simulink model "EPT"  (R2019b)
settings: Solver=FixedStepDiscrete  StartTime=0.0  StopTime=5  FixedStep=0.005  RelTol=1e-3  EnableMultiTasking=on
PreLoadFcn:
  | try, model_open; catch, disp('Error occurred while executing model pre-load callback: model_open.m'); disp('Please assure that the MATLAB working directory is set to the model directory before opening.'); end
InitFcn:
  | try, model_open; catch, end
undefined symbols (not defined in the file or in its folder): Bridge, GCM, H, ln, raptor_get_param_eval, raptor_get_safe_string, raptor_xcp_function
libraries: Raptor_lib x2810, simulink x374, hdlsllib x19
(part 40 of 45)

== system EPT/Foreground_TimeBase_5ms/CAN/CAN3_exec/PWCU_GENERATOR/PWCU/PWCU3_Tx3/Convert_Data2Byte ==
  Data : Inport
  Factor : Inport  Port=2
  Offset : Inport  Port=3
  Add1 : Sum
  Bitwise Operator : simulink/Logic and Bit Operations/Bitwise Operator  logicop=AND  UseBitMask=on  BitMask=bin2dec('1111111100000000')  BitMaskRealWorld=Stored Integer
  Bitwise Operator1 : simulink/Logic and Bit Operations/Bitwise Operator  logicop=AND  UseBitMask=on  BitMask=bin2dec('0000000011111111')  BitMaskRealWorld=Stored Integer
  Constant : Constant
  Data Type Conversion1 : DataTypeConversion  OutDataTypeStr=uint16
  Divide1 : Product  Inputs=*/
  Divide2 : Product  Inputs=**
  Shift Arithmetic : ArithShift  BitShiftNumber=8  BitShiftDirection=Right
  HighByte : Outport  VectorParamsAs1DForOutWhenUnconnected=off
  LowByte : Outport  Port=2  VectorParamsAs1DForOutWhenUnconnected=off
  wires:
  Constant/1 -> Divide1/1
  Divide1/1 -> Divide2/2
  Factor/1 -> Divide1/2
  Bitwise Operator/1 -> Shift Arithmetic/1
  Offset/1 -> Add1/2
  Shift Arithmetic/1 -> HighByte/1
  Bitwise Operator1/1 -> LowByte/1
  Data Type Conversion1/1 -> Bitwise Operator/1, Bitwise Operator1/1
  Add1/1 -> Divide2/1
  Data/1 -> Add1/1
  Divide2/1 -> Data Type Conversion1/1

== system EPT/Foreground_TimeBase_5ms/CAN/CAN3_exec/PWCU_GENERATOR/PWCU/PWCU3_Tx3/Convert_Data2Byte1 ==
  Data : Inport
  Factor : Inport  Port=2
  Offset : Inport  Port=3
  Add1 : Sum
  Bitwise Operator : simulink/Logic and Bit Operations/Bitwise Operator  logicop=AND  UseBitMask=on  BitMask=bin2dec('1111111100000000')  BitMaskRealWorld=Stored Integer
  Bitwise Operator1 : simulink/Logic and Bit Operations/Bitwise Operator  logicop=AND  UseBitMask=on  BitMask=bin2dec('0000000011111111')  BitMaskRealWorld=Stored Integer
  Constant : Constant
  Data Type Conversion1 : DataTypeConversion  OutDataTypeStr=uint16
  Divide1 : Product  Inputs=*/
  Divide2 : Product  Inputs=**
  Shift Arithmetic : ArithShift  BitShiftNumber=8  BitShiftDirection=Right
  HighByte : Outport  VectorParamsAs1DForOutWhenUnconnected=off
  LowByte : Outport  Port=2  VectorParamsAs1DForOutWhenUnconnected=off
  wires:
  Constant/1 -> Divide1/1
  Divide1/1 -> Divide2/2
  Factor/1 -> Divide1/2
  Bitwise Operator/1 -> Shift Arithmetic/1
  Offset/1 -> Add1/2
  Shift Arithmetic/1 -> HighByte/1
  Bitwise Operator1/1 -> LowByte/1
  Data Type Conversion1/1 -> Bitwise Operator/1, Bitwise Operator1/1
  Add1/1 -> Divide2/1
  Data/1 -> Add1/1
  Divide2/1 -> Data Type Conversion1/1

== system EPT/Foreground_TimeBase_5ms/CAN/CAN3_exec/PWCU_GENERATOR/PWCU/Subsystem/Cmd_PWCU_Current_PI  ==
  PWCU1_Cout : Inport
  PWCU2_Cout : Inport  Port=2
  PWCU3_Cout : Inport  Port=3
  Ipwcu1_cc_exp : Inport  Port=4
  Ipwcu2_cc_exp : Inport  Port=5
  Ipwcu3_cc_exp : Inport  Port=6
  Enable : EnablePort
  Constant : Constant  Value=-inf
  Demux : Demux  Outputs=3
  Mux : Mux  Inputs=3
  Product : Product
  Product1 : Product
  Saturation Dynamic1 : simulink/Discontinuities/Saturation Dynamic  OutMin=[]  OutMax=[]  OutDataTypeStr=Inherit: Same as second input  OutDataType=fixdt(1, 16)  OutScaling=2^-10  DoSatur=off
  Saturation Dynamic2 : simulink/Discontinuities/Saturation Dynamic  OutMin=[]  OutMax=[]  OutDataTypeStr=Inherit: Same as second input  OutDataType=fixdt(1, 16)  OutScaling=2^-10  DoSatur=off
  Sum : Sum  Inputs=+-
  Sum1 : Sum  Inputs=+++
  Sum2 : Sum  Inputs=+-
  Sum3 : Sum  Inputs=+-
  raptor_adjustment2 : Raptor_lib/Data Storage/raptor_adjustment  paramName='Cal_PWCU_PID_KP'  nameSource=Parameter  initValue=0.5  dataType=double  storage=Calibration  calDispType=Number  calEnum={'False', 'True'}  calGain=1.0  calOffset=0.0  calMax=inf  calMin=-inf  calFormat='-1'  calUnit=''  calHelp=''  calAccess=1  calFunction=raptor_xcp_function(gcb)  calDispHeaders=off  calColHeaders={'Col1' 'Col2' 'Col3'}  calRowHeaders={'Row1' 'Row2' 'Row3'}
      settings: SourceProductName=Raptor
  raptor_adjustment4 : Raptor_lib/Data Storage/raptor_adjustment  paramName='Cal_PWCU_PID_KI'  nameSource=Parameter  initValue=0.2  dataType=double  storage=Calibration  calDispType=Number  calEnum={'False', 'True'}  calGain=1.0  calOffset=0.0  calMax=inf  calMin=-inf  calFormat='-1'  calUnit=''  calHelp=''  calAccess=1  calFunction=raptor_xcp_function(gcb)  calDispHeaders=off  calColHeaders={'Col1' 'Col2' 'Col3'}  calRowHeaders={'Row1' 'Row2' 'Row3'}
      settings: SourceProductName=Raptor
  PWCU1_Cout_Cmd : Outport  VectorParamsAs1DForOutWhenUnconnected=off
  PWCU2_Cout_Cmd : Outport  Port=2  VectorParamsAs1DForOutWhenUnconnected=off
  PWCU3_Cout_Cmd : Outport  Port=3  VectorParamsAs1DForOutWhenUnconnected=off
  wires:
  Constant/1 -> Saturation Dynamic2/3, Saturation Dynamic1/3
  raptor_adjustment4/1 -> Saturation Dynamic2/1, Product1/1
  Product/1 -> Saturation Dynamic1/2
  Saturation Dynamic1/1 -> Sum1/1
  Saturation Dynamic2/1 -> Sum1/2
  PWCU1_Cout/1 -> Sum/2
  Ipwcu1_cc_exp/1 -> Sum/1
  Product1/1 -> Saturation Dynamic2/2
  raptor_adjustment2/1 -> Saturation Dynamic1/1, Product/1
  Ipwcu2_cc_exp/1 -> Sum2/1
  PWCU2_Cout/1 -> Sum2/2
  Ipwcu3_cc_exp/1 -> Sum3/1
  PWCU3_Cout/1 -> Sum3/2
  Sum/1 -> Mux/1
  Sum2/1 -> Mux/2
  Sum3/1 -> Mux/3
  Mux/1 -> Sum1/3, Product1/2, Product/2
  Demux/2 -> PWCU2_Cout_Cmd/1
  Demux/1 -> PWCU1_Cout_Cmd/1
  Demux/3 -> PWCU3_Cout_Cmd/1
  Sum1/1 -> Demux/1

== system EPT/Foreground_TimeBase_5ms/CAN/CAN3_exec/PWCU_GENERATOR/PWCU/Subsystem/CountTrigger2 ==
  Counter : Inport
  Constant1 : Constant  Value=0
  Constant3 : Constant
  CycleTrigger : Subsystem
  Switch : Switch  Threshold=1
  Unit Delay : UnitDelay  SampleTime=-1  HasFrameUpgradeWarning=on
  Tirgger : Outport  VectorParamsAs1DForOutWhenUnconnected=off
  wires:
  Switch/1 -> CycleTrigger/1(In1)
  Constant3/1 -> Switch/3
  Constant1/1 -> Switch/1
  Counter/1 -> CycleTrigger/2(In2)
  CycleTrigger/1(Trigger) -> Tirgger/1, Unit Delay/1
  Unit Delay/1 -> Switch/2

== system EPT/Foreground_TimeBase_5ms/CAN/CAN3_exec/PWCU_GENERATOR/PWCU/Subsystem/Latch3 ==
  Latch : Inport
  Reset : Inport  Port=2
  Switch1 : Switch  Criteria=u2 > Threshold
  Switch3 : Switch  Criteria=u2 > Threshold
  Unit Delay1 : UnitDelay  SampleTime=-1  HasFrameUpgradeWarning=on
  Output : Outport  VectorParamsAs1DForOutWhenUnconnected=off
  wires:
  Unit Delay1/1 -> Switch1/3
  Switch3/1 -> Output/1, Unit Delay1/1
  Reset/1 -> Switch3/2
  Latch/1 -> Switch1/1, Switch1/2
  Switch1/1 -> Switch3/3

== system EPT/Foreground_TimeBase_5ms/CAN/CAN3_exec/PWCU_GENERATOR/PWCU/Subsystem/Latch4 ==
  Latch : Inport
  Reset : Inport  Port=2
  Switch1 : Switch  Criteria=u2 > Threshold
  Switch3 : Switch  Criteria=u2 > Threshold
  Unit Delay1 : UnitDelay  SampleTime=-1  HasFrameUpgradeWarning=on
  Output : Outport  VectorParamsAs1DForOutWhenUnconnected=off
  wires:
  Switch1/1 -> Switch3/3
  Latch/1 -> Switch1/2, Switch1/1
  Reset/1 -> Switch3/2
  Switch3/1 -> Unit Delay1/1, Output/1
  Unit Delay1/1 -> Switch1/3

== system EPT/Foreground_TimeBase_5ms/CAN/CAN3_exec/PWCU_GENERATOR/PWCU/Subsystem/Latch5 ==
  Latch : Inport
  Reset : Inport  Port=2
  Switch1 : Switch  Criteria=u2 > Threshold
  Switch3 : Switch  Criteria=u2 > Threshold
  Unit Delay1 : UnitDelay  SampleTime=-1  HasFrameUpgradeWarning=on
  Output : Outport  VectorParamsAs1DForOutWhenUnconnected=off
  wires:
  Switch1/1 -> Switch3/3
  Latch/1 -> Switch1/2, Switch1/1
  Reset/1 -> Switch3/2
  Switch3/1 -> Unit Delay1/1, Output/1
  Unit Delay1/1 -> Switch1/3

== system EPT/Foreground_TimeBase_5ms/CAN/CAN3_exec/SEVCON_MCU /SEVCON_TX_0X210_20ms /Delay/CycleTrigger ==
  In1 : Inport
  In2 : Inport  Port=2
  Add : Sum
  Add2 : Sum  Inputs=+-
  Constant2 : Constant  Value=0
  Constant3 : Constant
  Data Type Conversion1 : DataTypeConversion
  Data Type Conversion2 : DataTypeConversion
  Relational Operator1 : RelationalOperator  OutDataTypeStr=boolean  RndMeth=Simplest
  Saturation : Saturate  UpperLimit=inf  LowerLimit=2
  Switch : Switch  Threshold=1
  Unit Delay : UnitDelay  SampleTime=-1  HasFrameUpgradeWarning=on
  Trigger : Outport  VectorParamsAs1DForOutWhenUnconnected=off
  wires:
  Constant3/1 -> Add2/2
  In2/1 -> Saturation/1
  Add2/1 -> Data Type Conversion1/1
  Data Type Conversion2/1 -> Switch/2, Add/2
  Constant2/1 -> Switch/3
  Data Type Conversion1/1 -> Relational Operator1/2
  Relational Operator1/1 -> Trigger/1
  Switch/1 -> Unit Delay/1, Relational Operator1/1
  Unit Delay/1 -> Add/1
  In1/1 -> Data Type Conversion2/1
  Add/1 -> Switch/1
  Saturation/1 -> Add2/1

== system EPT/Foreground_TimeBase_5ms/CAN/CAN3_exec/SEVCON_MCU /SEVCON_TX_0X210_20ms /Delay1/CycleTrigger ==
  In1 : Inport
  In2 : Inport  Port=2
  Add : Sum
  Add2 : Sum  Inputs=+-
  Constant2 : Constant  Value=0
  Constant3 : Constant
  Data Type Conversion1 : DataTypeConversion
  Data Type Conversion2 : DataTypeConversion
  Relational Operator1 : RelationalOperator  OutDataTypeStr=boolean  RndMeth=Simplest
  Saturation : Saturate  UpperLimit=inf  LowerLimit=2
  Switch : Switch  Threshold=1
  Unit Delay : UnitDelay  SampleTime=-1  HasFrameUpgradeWarning=on
  Trigger : Outport  VectorParamsAs1DForOutWhenUnconnected=off
  wires:
  Constant3/1 -> Add2/2
  In2/1 -> Saturation/1
  Add2/1 -> Data Type Conversion1/1
  Data Type Conversion2/1 -> Switch/2, Add/2
  Constant2/1 -> Switch/3
  Data Type Conversion1/1 -> Relational Operator1/2
  Relational Operator1/1 -> Trigger/1
  Switch/1 -> Unit Delay/1, Relational Operator1/1
  Unit Delay/1 -> Add/1
  In1/1 -> Data Type Conversion2/1
  Add/1 -> Switch/1
  Saturation/1 -> Add2/1

== system EPT/Foreground_TimeBase_5ms/CAN/CAN3_exec/SEVCON_MCU /SEVCON_TX_0X210_20ms /Delay3/CycleTrigger ==
  In1 : Inport
  In2 : Inport  Port=2
  Add : Sum
  Add2 : Sum  Inputs=+-
  Constant2 : Constant  Value=0
  Constant3 : Constant
  Data Type Conversion1 : DataTypeConversion
  Data Type Conversion2 : DataTypeConversion
  Relational Operator1 : RelationalOperator  OutDataTypeStr=boolean  RndMeth=Simplest
  Saturation : Saturate  UpperLimit=inf  LowerLimit=2
  Switch : Switch  Threshold=1
  Unit Delay : UnitDelay  SampleTime=-1  HasFrameUpgradeWarning=on
  Trigger : Outport  VectorParamsAs1DForOutWhenUnconnected=off
  wires:
  Saturation/1 -> Add2/1
  Add/1 -> Switch/1
  In1/1 -> Data Type Conversion2/1
  Unit Delay/1 -> Add/1
  Switch/1 -> Relational Operator1/1, Unit Delay/1
  Relational Operator1/1 -> Trigger/1
  Data Type Conversion1/1 -> Relational Operator1/2
  Constant2/1 -> Switch/3
  Data Type Conversion2/1 -> Add/2, Switch/2
  Add2/1 -> Data Type Conversion1/1
  In2/1 -> Saturation/1
  Constant3/1 -> Add2/2

== system EPT/Foreground_TimeBase_5ms/CAN/CAN3_exec/SWCU/EPT to SWCU Enable Control/Delay/CycleTrigger ==
  In1 : Inport
  In2 : Inport  Port=2
  Add : Sum
  Add1 : Sum
  Add2 : Sum  Inputs=+-
  Constant1 : Constant
  Constant2 : Constant  Value=0
  Constant3 : Constant
  Data Type Conversion1 : DataTypeConversion
  Data Type Conversion2 : DataTypeConversion
  Display : Display
  Relational Operator1 : RelationalOperator  OutDataTypeStr=boolean  RndMeth=Simplest
  Saturation : Saturate  UpperLimit=inf  LowerLimit=2
  Scope : Scope
  Scope1 : Scope
  Scope2 : Scope
  Switch : Switch  Threshold=1
  Unit Delay : UnitDelay  SampleTime=-1  HasFrameUpgradeWarning=on
  Unit Delay1 : UnitDelay  SampleTime=-1  HasFrameUpgradeWarning=on
  Trigger : Outport  VectorParamsAs1DForOutWhenUnconnected=off
  wires:
  Saturation/1 -> Add2/1
  Add/1 -> Switch/1
  In1/1 -> Data Type Conversion2/1
  Unit Delay/1 -> Add/1
  Switch/1 -> Relational Operator1/1, Scope1/1, Unit Delay/1
  Add1/1 -> Scope/1, Unit Delay1/1, Display/1
  Unit Delay1/1 -> Add1/1
  Constant1/1 -> Add1/2
  Relational Operator1/1 -> Scope2/1, Trigger/1
  Data Type Conversion1/1 -> Relational Operator1/2
  Constant2/1 -> Switch/3
  Data Type Conversion2/1 -> Add/2, Switch/2
  Add2/1 -> Data Type Conversion1/1
  In2/1 -> Saturation/1
  Constant3/1 -> Add2/2

== system EPT/Foreground_TimeBase_5ms/CHG//DCHG_PW_Control/Coulomb Counting Algorithm/Coulomb Counting Algorithm/20ms/CountTrigger3/CycleTrigger ==
  In1 : Inport
  In2 : Inport  Port=2
  Add : Sum
  Add2 : Sum  Inputs=+-
  Constant2 : Constant  Value=0
  Constant3 : Constant
  Data Type Conversion1 : DataTypeConversion
  Data Type Conversion2 : DataTypeConversion
  Relational Operator1 : RelationalOperator  OutDataTypeStr=boolean  RndMeth=Simplest
  Scope1 : Scope
  Scope2 : Scope
  Switch : Switch  Threshold=1
  Unit Delay : UnitDelay  SampleTime=-1  HasFrameUpgradeWarning=on
  Trigger : Outport  VectorParamsAs1DForOutWhenUnconnected=off
  wires:
  Constant3/1 -> Add2/2
  In2/1 -> Add2/1
  Add2/1 -> Data Type Conversion1/1
  Data Type Conversion2/1 -> Switch/2, Add/2
  Constant2/1 -> Switch/3
  Data Type Conversion1/1 -> Relational Operator1/2
  Relational Operator1/1 -> Trigger/1, Scope2/1
  Switch/1 -> Unit Delay/1, Scope1/1, Relational Operator1/1
  Unit Delay/1 -> Add/1
  In1/1 -> Data Type Conversion2/1
  Add/1 -> Switch/1

== system EPT/Foreground_TimeBase_5ms/CHG//DCHG_PW_Control/Coulomb Counting Algorithm/WH /20ms/CountTrigger3/CycleTrigger ==
  In1 : Inport
  In2 : Inport  Port=2
  Add : Sum
  Add2 : Sum  Inputs=+-
  Constant2 : Constant  Value=0
  Constant3 : Constant
  Data Type Conversion1 : DataTypeConversion
  Data Type Conversion2 : DataTypeConversion
  Relational Operator1 : RelationalOperator  OutDataTypeStr=boolean  RndMeth=Simplest
  Scope1 : Scope
  Scope2 : Scope
  Switch : Switch  Threshold=1
  Unit Delay : UnitDelay  SampleTime=-1  HasFrameUpgradeWarning=on
  Trigger : Outport  VectorParamsAs1DForOutWhenUnconnected=off
  wires:
  Add/1 -> Switch/1
  In1/1 -> Data Type Conversion2/1
  Unit Delay/1 -> Add/1
  Switch/1 -> Relational Operator1/1, Scope1/1, Unit Delay/1
  Relational Operator1/1 -> Scope2/1, Trigger/1
  Data Type Conversion1/1 -> Relational Operator1/2
  Constant2/1 -> Switch/3
  Data Type Conversion2/1 -> Add/2, Switch/2
  Add2/1 -> Data Type Conversion1/1
  In2/1 -> Add2/1
  Constant3/1 -> Add2/2

== system EPT/Foreground_TimeBase_5ms/CHG//DCHG_PW_Control/Enhanced Coulomb Counting Algorithm/Coulomb Counting/20ms/CountTrigger3/CycleTrigger ==
  In1 : Inport
  In2 : Inport  Port=2
  Add : Sum
  Add2 : Sum  Inputs=+-
  Constant2 : Constant  Value=0
  Constant3 : Constant
  Data Type Conversion1 : DataTypeConversion
  Data Type Conversion2 : DataTypeConversion
  Relational Operator1 : RelationalOperator  OutDataTypeStr=boolean  RndMeth=Simplest
  Scope1 : Scope
  Scope2 : Scope
  Switch : Switch  Threshold=1
  Unit Delay : UnitDelay  SampleTime=-1  HasFrameUpgradeWarning=on
  Trigger : Outport  VectorParamsAs1DForOutWhenUnconnected=off
  wires:
  Add/1 -> Switch/1
  In1/1 -> Data Type Conversion2/1
  Unit Delay/1 -> Add/1
  Switch/1 -> Relational Operator1/1, Scope1/1, Unit Delay/1
  Relational Operator1/1 -> Scope2/1, Trigger/1
  Data Type Conversion1/1 -> Relational Operator1/2
  Constant2/1 -> Switch/3
  Data Type Conversion2/1 -> Add/2, Switch/2
  Add2/1 -> Data Type Conversion1/1
  In2/1 -> Add2/1
  Constant3/1 -> Add2/2

== system EPT/Foreground_TimeBase_5ms/CHG//DCHG_PW_Control/Enhanced Coulomb Counting Algorithm Backup/Coulomb Counting1/20ms/CountTrigger3/CycleTrigger ==
  In1 : Inport
  In2 : Inport  Port=2
  Add : Sum
  Add2 : Sum  Inputs=+-
  Constant2 : Constant  Value=0
  Constant3 : Constant
  Data Type Conversion1 : DataTypeConversion
  Data Type Conversion2 : DataTypeConversion
  Relational Operator1 : RelationalOperator  OutDataTypeStr=boolean  RndMeth=Simplest
  Scope1 : Scope
  Scope2 : Scope
  Switch : Switch  Threshold=1
  Unit Delay : UnitDelay  SampleTime=-1  HasFrameUpgradeWarning=on
  Trigger : Outport  VectorParamsAs1DForOutWhenUnconnected=off
  wires:
  Constant3/1 -> Add2/2
  In2/1 -> Add2/1
  Add2/1 -> Data Type Conversion1/1
  Data Type Conversion2/1 -> Switch/2, Add/2
  Constant2/1 -> Switch/3
  Data Type Conversion1/1 -> Relational Operator1/2
  Relational Operator1/1 -> Trigger/1, Scope2/1
  Switch/1 -> Unit Delay/1, Scope1/1, Relational Operator1/1
  Unit Delay/1 -> Add/1
  In1/1 -> Data Type Conversion2/1
  Add/1 -> Switch/1

== system EPT/Foreground_TimeBase_5ms/E//W /BP-OBU_E//W/BP-OBU_E//W/BP-OBU_Fault_G4/Fault CMU CAN ID/Delay34 ==
  Condition : Inport
  TimeCount : Inport  Port=2
  Constant10 : Constant
  Constant11 : Constant  Value=0
  Constant8 : Constant  Value=0
  CycleTrigger : Subsystem
  Switch2 : Switch  Threshold=1
  Switch3 : Switch  Threshold=1
  Unit Delay1 : UnitDelay  SampleTime=-1  HasFrameUpgradeWarning=on
  Unit Delay2 : UnitDelay  SampleTime=-1  HasFrameUpgradeWarning=on
  Output : Outport  VectorParamsAs1DForOutWhenUnconnected=off
  wires:
  TimeCount/1 -> CycleTrigger/2(In2)
  Condition/1 -> Switch3/2
  CycleTrigger/1(Trigger) -> Switch2/2, Unit Delay1/1
  Constant8/1 -> Switch2/1
  Constant10/1 -> Switch2/3
  Switch3/1 -> CycleTrigger/1(In1)
  Constant11/1 -> Switch3/3
  Unit Delay2/1 -> Switch3/1
  Switch2/1 -> Unit Delay2/1
  Unit Delay1/1 -> Output/1

== system EPT/Foreground_TimeBase_5ms/E//W /BP-OBU_E//W/BP-OBU_E//W/BP-OBU_Fault_G4/Fault CMU CAN ID/Delay35 ==
  Condition : Inport
  TimeCount : Inport  Port=2
  Constant10 : Constant
  Constant11 : Constant  Value=0
  Constant8 : Constant  Value=0
  CycleTrigger : Subsystem
  Switch2 : Switch  Threshold=1
  Switch3 : Switch  Threshold=1
  Unit Delay1 : UnitDelay  SampleTime=-1  HasFrameUpgradeWarning=on
  Unit Delay2 : UnitDelay  SampleTime=-1  HasFrameUpgradeWarning=on
  Output : Outport  VectorParamsAs1DForOutWhenUnconnected=off
  wires:
  Unit Delay1/1 -> Output/1
  Switch2/1 -> Unit Delay2/1
  Unit Delay2/1 -> Switch3/1
  Constant11/1 -> Switch3/3
  Switch3/1 -> CycleTrigger/1(In1)
  Constant10/1 -> Switch2/3
  Constant8/1 -> Switch2/1
  CycleTrigger/1(Trigger) -> Unit Delay1/1, Switch2/2
  Condition/1 -> Switch3/2
  TimeCount/1 -> CycleTrigger/2(In2)

== system EPT/Foreground_TimeBase_5ms/E//W /BP-OBU_E//W/BP-OBU_E//W/BP-OBU_Fault_G4/Fault CMU CAN ID/Latch39 ==
  Latch : Inport
  Reset : Inport  Port=2
  Switch1 : Switch  Criteria=u2 > Threshold
  Switch3 : Switch  Criteria=u2 > Threshold
  Unit Delay1 : UnitDelay  SampleTime=-1  HasFrameUpgradeWarning=on
  Output : Outport  VectorParamsAs1DForOutWhenUnconnected=off
  wires:
  Unit Delay1/1 -> Switch1/3
  Switch3/1 -> Output/1, Unit Delay1/1
  Reset/1 -> Switch3/2
  Latch/1 -> Switch1/1, Switch1/2
  Switch1/1 -> Switch3/3

== system EPT/Foreground_TimeBase_5ms/E//W /BP-OBU_E//W/BP-OBU_E//W/BP-OBU_Fault_G4/Fault CMU CAN ID/Latch40 ==
  Latch : Inport
  Reset : Inport  Port=2
  Switch1 : Switch  Criteria=u2 > Threshold
  Switch3 : Switch  Criteria=u2 > Threshold
  Unit Delay1 : UnitDelay  SampleTime=-1  HasFrameUpgradeWarning=on
  Output : Outport  VectorParamsAs1DForOutWhenUnconnected=off
  wires:
  Switch1/1 -> Switch3/3
  Latch/1 -> Switch1/2, Switch1/1
  Reset/1 -> Switch3/2
  Switch3/1 -> Unit Delay1/1, Output/1
  Unit Delay1/1 -> Switch1/3

== system EPT/Foreground_TimeBase_5ms/E//W /BP-OBU_E//W/BP-OBU_E//W/BP-OBU_Warning//Fault_G1/Internal Res E//W/Delay4 ==
  Condition : Inport
  TimeCount : Inport  Port=2
  Constant10 : Constant
  Constant11 : Constant  Value=0
  Constant8 : Constant  Value=0
  CycleTrigger : Subsystem
  Switch2 : Switch  Threshold=1
  Switch3 : Switch  Threshold=1
  Unit Delay1 : UnitDelay  SampleTime=-1  HasFrameUpgradeWarning=on
  Unit Delay2 : UnitDelay  SampleTime=-1  HasFrameUpgradeWarning=on
  Output : Outport  VectorParamsAs1DForOutWhenUnconnected=off
  wires:
  TimeCount/1 -> CycleTrigger/2(In2)
  Condition/1 -> Switch3/2
  CycleTrigger/1(Trigger) -> Switch2/2, Unit Delay1/1
  Constant8/1 -> Switch2/1
  Constant10/1 -> Switch2/3
  Switch3/1 -> CycleTrigger/1(In1)
  Constant11/1 -> Switch3/3
  Unit Delay2/1 -> Switch3/1
  Switch2/1 -> Unit Delay2/1
  Unit Delay1/1 -> Output/1

== system EPT/Foreground_TimeBase_5ms/E//W /BP-OBU_E//W/BP-OBU_E//W/BP-OBU_Warning//Fault_G1/Internal Res E//W/Delay5 ==
  Condition : Inport
  TimeCount : Inport  Port=2
  Constant10 : Constant
  Constant11 : Constant  Value=0
  Constant8 : Constant  Value=0
  CycleTrigger : Subsystem
  Switch2 : Switch  Threshold=1
  Switch3 : Switch  Threshold=1
  Unit Delay1 : UnitDelay  SampleTime=-1  HasFrameUpgradeWarning=on
  Unit Delay2 : UnitDelay  SampleTime=-1  HasFrameUpgradeWarning=on
  Output : Outport  VectorParamsAs1DForOutWhenUnconnected=off
  wires:
  Unit Delay1/1 -> Output/1
  Switch2/1 -> Unit Delay2/1
  Unit Delay2/1 -> Switch3/1
  Constant11/1 -> Switch3/3
  Switch3/1 -> CycleTrigger/1(In1)
  Constant10/1 -> Switch2/3
  Constant8/1 -> Switch2/1
  CycleTrigger/1(Trigger) -> Unit Delay1/1, Switch2/2
  Condition/1 -> Switch3/2
  TimeCount/1 -> CycleTrigger/2(In2)

== system EPT/Foreground_TimeBase_5ms/E//W /BP-OBU_E//W/BP-OBU_E//W/BP-OBU_Warning//Fault_G1/Internal Res E//W/Delay6 ==
  Condition : Inport
  TimeCount : Inport  Port=2
  Constant10 : Constant
  Constant11 : Constant  Value=0
  Constant8 : Constant  Value=0
  CycleTrigger : Subsystem
  Switch2 : Switch  Threshold=1
  Switch3 : Switch  Threshold=1
  Unit Delay1 : UnitDelay  SampleTime=-1  HasFrameUpgradeWarning=on
  Unit Delay2 : UnitDelay  SampleTime=-1  HasFrameUpgradeWarning=on
  Output : Outport  VectorParamsAs1DForOutWhenUnconnected=off
  wires:
  TimeCount/1 -> CycleTrigger/2(In2)
  Condition/1 -> Switch3/2
  CycleTrigger/1(Trigger) -> Switch2/2, Unit Delay1/1
  Constant8/1 -> Switch2/1
  Constant10/1 -> Switch2/3
  Switch3/1 -> CycleTrigger/1(In1)
  Constant11/1 -> Switch3/3
  Unit Delay2/1 -> Switch3/1
  Switch2/1 -> Unit Delay2/1
  Unit Delay1/1 -> Output/1

== system EPT/Foreground_TimeBase_5ms/E//W /BP-OBU_E//W/BP-OBU_E//W/BP-OBU_Warning//Fault_G1/Internal Res E//W/Delay7 ==
  Condition : Inport
  TimeCount : Inport  Port=2
  Constant10 : Constant
  Constant11 : Constant  Value=0
  Constant8 : Constant  Value=0
  CycleTrigger : Subsystem
  Switch2 : Switch  Threshold=1
  Switch3 : Switch  Threshold=1
  Unit Delay1 : UnitDelay  SampleTime=-1  HasFrameUpgradeWarning=on
  Unit Delay2 : UnitDelay  SampleTime=-1  HasFrameUpgradeWarning=on
  Output : Outport  VectorParamsAs1DForOutWhenUnconnected=off
  wires:
  Unit Delay1/1 -> Output/1
  Switch2/1 -> Unit Delay2/1
  Unit Delay2/1 -> Switch3/1
  Constant11/1 -> Switch3/3
  Switch3/1 -> CycleTrigger/1(In1)
  Constant10/1 -> Switch2/3
  Constant8/1 -> Switch2/1
  CycleTrigger/1(Trigger) -> Unit Delay1/1, Switch2/2
  Condition/1 -> Switch3/2
  TimeCount/1 -> CycleTrigger/2(In2)

== system EPT/Foreground_TimeBase_5ms/E//W /BP-OBU_E//W/BP-OBU_E//W/BP-OBU_Warning//Fault_G1/Internal Res E//W/Delay8 ==
  Condition : Inport
  TimeCount : Inport  Port=2
  Constant10 : Constant
  Constant11 : Constant  Value=0
  Constant8 : Constant  Value=0
  CycleTrigger : Subsystem
  Switch2 : Switch  Threshold=1
  Switch3 : Switch  Threshold=1
  Unit Delay1 : UnitDelay  SampleTime=-1  HasFrameUpgradeWarning=on
  Unit Delay2 : UnitDelay  SampleTime=-1  HasFrameUpgradeWarning=on
  Output : Outport  VectorParamsAs1DForOutWhenUnconnected=off
  wires:
  TimeCount/1 -> CycleTrigger/2(In2)
  Condition/1 -> Switch3/2
  CycleTrigger/1(Trigger) -> Switch2/2, Unit Delay1/1
  Constant8/1 -> Switch2/1
  Constant10/1 -> Switch2/3
  Switch3/1 -> CycleTrigger/1(In1)
  Constant11/1 -> Switch3/3
  Unit Delay2/1 -> Switch3/1
  Switch2/1 -> Unit Delay2/1
  Unit Delay1/1 -> Output/1

== system EPT/Foreground_TimeBase_5ms/E//W /BP-OBU_E//W/BP-OBU_E//W/BP-OBU_Warning//Fault_G1/Internal Res E//W/Delay9 ==
  Condition : Inport
  TimeCount : Inport  Port=2
  Constant10 : Constant
  Constant11 : Constant  Value=0
  Constant8 : Constant  Value=0
  CycleTrigger : Subsystem
  Switch2 : Switch  Threshold=1
  Switch3 : Switch  Threshold=1
  Unit Delay1 : UnitDelay  SampleTime=-1  HasFrameUpgradeWarning=on
  Unit Delay2 : UnitDelay  SampleTime=-1  HasFrameUpgradeWarning=on
  Output : Outport  VectorParamsAs1DForOutWhenUnconnected=off
  wires:
  Unit Delay1/1 -> Output/1
  Switch2/1 -> Unit Delay2/1
  Unit Delay2/1 -> Switch3/1
  Constant11/1 -> Switch3/3
  Switch3/1 -> CycleTrigger/1(In1)
  Constant10/1 -> Switch2/3
  Constant8/1 -> Switch2/1
  CycleTrigger/1(Trigger) -> Unit Delay1/1, Switch2/2
  Condition/1 -> Switch3/2
  TimeCount/1 -> CycleTrigger/2(In2)

== system EPT/Foreground_TimeBase_5ms/E//W /BP-OBU_E//W/BP-OBU_E//W/BP-OBU_Warning//Fault_G1/Internal Res E//W/Latch1 ==
  Latch : Inport
  Reset : Inport  Port=2
  Switch1 : Switch  Criteria=u2 > Threshold
  Switch3 : Switch  Criteria=u2 > Threshold
  Unit Delay1 : UnitDelay  SampleTime=-1  HasFrameUpgradeWarning=on
  Output : Outport  VectorParamsAs1DForOutWhenUnconnected=off
  wires:
  Unit Delay1/1 -> Switch1/3
  Switch3/1 -> Output/1, Unit Delay1/1
  Reset/1 -> Switch3/2
  Latch/1 -> Switch1/1, Switch1/2
  Switch1/1 -> Switch3/3

== system EPT/Foreground_TimeBase_5ms/E//W /BP-OBU_E//W/BP-OBU_E//W/BP-OBU_Warning//Fault_G1/Internal Res E//W/Latch2 ==
  Latch : Inport
  Reset : Inport  Port=2
  Switch1 : Switch  Criteria=u2 > Threshold
  Switch3 : Switch  Criteria=u2 > Threshold
  Unit Delay1 : UnitDelay  SampleTime=-1  HasFrameUpgradeWarning=on
  Output : Outport  VectorParamsAs1DForOutWhenUnconnected=off
  wires:
  Unit Delay1/1 -> Switch1/3
  Switch3/1 -> Output/1, Unit Delay1/1
  Reset/1 -> Switch3/2
  Latch/1 -> Switch1/1, Switch1/2
  Switch1/1 -> Switch3/3

== system EPT/Foreground_TimeBase_5ms/E//W /BP-OBU_E//W/BP-OBU_E//W/BP-OBU_Warning//Fault_G1/Internal Res E//W/Latch4 ==
  Latch : Inport
  Reset : Inport  Port=2
  Switch1 : Switch  Criteria=u2 > Threshold
  Switch3 : Switch  Criteria=u2 > Threshold
  Unit Delay1 : UnitDelay  SampleTime=-1  HasFrameUpgradeWarning=on
  Output : Outport  VectorParamsAs1DForOutWhenUnconnected=off
  wires:
  Unit Delay1/1 -> Switch1/3
  Switch3/1 -> Output/1, Unit Delay1/1
  Reset/1 -> Switch3/2
  Latch/1 -> Switch1/1, Switch1/2
  Switch1/1 -> Switch3/3

== system EPT/Foreground_TimeBase_5ms/E//W /BP-OBU_E//W/BP-OBU_E//W/BP-OBU_Warning//Fault_G1/Internal Res E//W/Latch5 ==
  Latch : Inport
  Reset : Inport  Port=2
  Switch1 : Switch  Criteria=u2 > Threshold
  Switch3 : Switch  Criteria=u2 > Threshold
  Unit Delay1 : UnitDelay  SampleTime=-1  HasFrameUpgradeWarning=on
  Output : Outport  VectorParamsAs1DForOutWhenUnconnected=off
  wires:
  Switch1/1 -> Switch3/3
  Latch/1 -> Switch1/2, Switch1/1
  Reset/1 -> Switch3/2
  Switch3/1 -> Unit Delay1/1, Output/1
  Unit Delay1/1 -> Switch1/3

== system EPT/Foreground_TimeBase_5ms/E//W /BP-OBU_E//W/BP-OBU_E//W/BP-OBU_Warning//Fault_G1/Internal Res E//W/Latch6 ==
  Latch : Inport
  Reset : Inport  Port=2
  Switch1 : Switch  Criteria=u2 > Threshold
  Switch3 : Switch  Criteria=u2 > Threshold
  Unit Delay1 : UnitDelay  SampleTime=-1  HasFrameUpgradeWarning=on
  Output : Outport  VectorParamsAs1DForOutWhenUnconnected=off
  wires:
  Unit Delay1/1 -> Switch1/3
  Switch3/1 -> Output/1, Unit Delay1/1
  Reset/1 -> Switch3/2
  Latch/1 -> Switch1/1, Switch1/2
  Switch1/1 -> Switch3/3

== system EPT/Foreground_TimeBase_5ms/E//W /BP-OBU_E//W/BP-OBU_E//W/BP-OBU_Warning//Fault_G1/Internal Res E//W/Latch7 ==
  Latch : Inport
  Reset : Inport  Port=2
  Switch1 : Switch  Criteria=u2 > Threshold
  Switch3 : Switch  Criteria=u2 > Threshold
  Unit Delay1 : UnitDelay  SampleTime=-1  HasFrameUpgradeWarning=on
  Output : Outport  VectorParamsAs1DForOutWhenUnconnected=off
  wires:
  Switch1/1 -> Switch3/3
  Latch/1 -> Switch1/2, Switch1/1
  Reset/1 -> Switch3/2
  Switch3/1 -> Unit Delay1/1, Output/1
  Unit Delay1/1 -> Switch1/3

== system EPT/Foreground_TimeBase_5ms/E//W /BP-OBU_E//W/BP-OBU_E//W/BP-OBU_Warning//Fault_G1/Internal Res E//W/Latch8 ==
  Latch : Inport
  Reset : Inport  Port=2
  Switch1 : Switch  Criteria=u2 > Threshold
  Switch3 : Switch  Criteria=u2 > Threshold
  Unit Delay1 : UnitDelay  SampleTime=-1  HasFrameUpgradeWarning=on
  Output : Outport  VectorParamsAs1DForOutWhenUnconnected=off
  wires:
  Unit Delay1/1 -> Switch1/3
  Switch3/1 -> Output/1, Unit Delay1/1
  Reset/1 -> Switch3/2
  Latch/1 -> Switch1/1, Switch1/2
  Switch1/1 -> Switch3/3

== system EPT/Foreground_TimeBase_5ms/E//W /BP-OBU_E//W/BP-OBU_E//W/BP-OBU_Warning//Fault_G1/Internal Res E//W/Latch9 ==
  Latch : Inport
  Reset : Inport  Port=2
  Switch1 : Switch  Criteria=u2 > Threshold
  Switch3 : Switch  Criteria=u2 > Threshold
  Unit Delay1 : UnitDelay  SampleTime=-1  HasFrameUpgradeWarning=on
  Output : Outport  VectorParamsAs1DForOutWhenUnconnected=off
  wires:
  Switch1/1 -> Switch3/3
  Latch/1 -> Switch1/2, Switch1/1
  Reset/1 -> Switch3/2
  Switch3/1 -> Unit Delay1/1, Output/1
  Unit Delay1/1 -> Switch1/3

== system EPT/Foreground_TimeBase_5ms/E//W /BP-OBU_E//W/BP-OBU_E//W/BP-OBU_Warning//Fault_G1/SOC E//W/Delay16 ==
  Condition : Inport
  TimeCount : Inport  Port=2
  Constant10 : Constant
  Constant11 : Constant  Value=0
  Constant8 : Constant  Value=0
  CycleTrigger : Subsystem
  Switch2 : Switch  Threshold=1
  Switch3 : Switch  Threshold=1
  Unit Delay1 : UnitDelay  SampleTime=-1  HasFrameUpgradeWarning=on
  Unit Delay2 : UnitDelay  SampleTime=-1  HasFrameUpgradeWarning=on
  Output : Outport  VectorParamsAs1DForOutWhenUnconnected=off
  wires:
  Unit Delay1/1 -> Output/1
  Switch2/1 -> Unit Delay2/1
  Unit Delay2/1 -> Switch3/1
  Constant11/1 -> Switch3/3
  Switch3/1 -> CycleTrigger/1(In1)
  Constant10/1 -> Switch2/3
  Constant8/1 -> Switch2/1
  CycleTrigger/1(Trigger) -> Unit Delay1/1, Switch2/2
  Condition/1 -> Switch3/2
  TimeCount/1 -> CycleTrigger/2(In2)

== system EPT/Foreground_TimeBase_5ms/E//W /BP-OBU_E//W/BP-OBU_E//W/BP-OBU_Warning//Fault_G1/SOC E//W/Delay17 ==
  Condition : Inport
  TimeCount : Inport  Port=2
  Constant10 : Constant
  Constant11 : Constant  Value=0
  Constant8 : Constant  Value=0
  CycleTrigger : Subsystem
  Switch2 : Switch  Threshold=1
  Switch3 : Switch  Threshold=1
  Unit Delay1 : UnitDelay  SampleTime=-1  HasFrameUpgradeWarning=on
  Unit Delay2 : UnitDelay  SampleTime=-1  HasFrameUpgradeWarning=on
  Output : Outport  VectorParamsAs1DForOutWhenUnconnected=off
  wires:
  TimeCount/1 -> CycleTrigger/2(In2)
  Condition/1 -> Switch3/2
  CycleTrigger/1(Trigger) -> Switch2/2, Unit Delay1/1
  Constant8/1 -> Switch2/1
  Constant10/1 -> Switch2/3
  Switch3/1 -> CycleTrigger/1(In1)
  Constant11/1 -> Switch3/3
  Unit Delay2/1 -> Switch3/1
  Switch2/1 -> Unit Delay2/1
  Unit Delay1/1 -> Output/1

== system EPT/Foreground_TimeBase_5ms/E//W /BP-OBU_E//W/BP-OBU_E//W/BP-OBU_Warning//Fault_G1/SOC E//W/Latch16 ==
  Latch : Inport
  Reset : Inport  Port=2
  Switch1 : Switch  Criteria=u2 > Threshold
  Switch3 : Switch  Criteria=u2 > Threshold
  Unit Delay1 : UnitDelay  SampleTime=-1  HasFrameUpgradeWarning=on
  Output : Outport  VectorParamsAs1DForOutWhenUnconnected=off
  wires:
  Switch1/1 -> Switch3/3
  Latch/1 -> Switch1/2, Switch1/1
  Reset/1 -> Switch3/2
  Switch3/1 -> Unit Delay1/1, Output/1
  Unit Delay1/1 -> Switch1/3

== system EPT/Foreground_TimeBase_5ms/E//W /BP-OBU_E//W/BP-OBU_E//W/BP-OBU_Warning//Fault_G1/SOC E//W/Latch17 ==
  Latch : Inport
  Reset : Inport  Port=2
  Switch1 : Switch  Criteria=u2 > Threshold
  Switch3 : Switch  Criteria=u2 > Threshold
  Unit Delay1 : UnitDelay  SampleTime=-1  HasFrameUpgradeWarning=on
  Output : Outport  VectorParamsAs1DForOutWhenUnconnected=off
  wires:
  Unit Delay1/1 -> Switch1/3
  Switch3/1 -> Output/1, Unit Delay1/1
  Reset/1 -> Switch3/2
  Latch/1 -> Switch1/1, Switch1/2
  Switch1/1 -> Switch3/3

== system EPT/Foreground_TimeBase_5ms/E//W /BP-OBU_E//W/BP-OBU_E//W/BP-OBU_Warning//Fault_G1/Tbp E//W/Delay10 ==
  Condition : Inport
  TimeCount : Inport  Port=2
  Constant10 : Constant
  Constant11 : Constant  Value=0
  Constant8 : Constant  Value=0
  CycleTrigger : Subsystem
  Switch2 : Switch  Threshold=1
  Switch3 : Switch  Threshold=1
  Unit Delay1 : UnitDelay  SampleTime=-1  HasFrameUpgradeWarning=on
  Unit Delay2 : UnitDelay  SampleTime=-1  HasFrameUpgradeWarning=on
  Output : Outport  VectorParamsAs1DForOutWhenUnconnected=off
  wires:
  TimeCount/1 -> CycleTrigger/2(In2)
  Condition/1 -> Switch3/2
  CycleTrigger/1(Trigger) -> Switch2/2, Unit Delay1/1
  Constant8/1 -> Switch2/1
  Constant10/1 -> Switch2/3
  Switch3/1 -> CycleTrigger/1(In1)
  Constant11/1 -> Switch3/3
  Unit Delay2/1 -> Switch3/1
  Switch2/1 -> Unit Delay2/1
  Unit Delay1/1 -> Output/1

== system EPT/Foreground_TimeBase_5ms/E//W /BP-OBU_E//W/BP-OBU_E//W/BP-OBU_Warning//Fault_G1/Tbp E//W/Delay11 ==
  Condition : Inport
  TimeCount : Inport  Port=2
  Constant10 : Constant
  Constant11 : Constant  Value=0
  Constant8 : Constant  Value=0
  CycleTrigger : Subsystem
  Switch2 : Switch  Threshold=1
  Switch3 : Switch  Threshold=1
  Unit Delay1 : UnitDelay  SampleTime=-1  HasFrameUpgradeWarning=on
  Unit Delay2 : UnitDelay  SampleTime=-1  HasFrameUpgradeWarning=on
  Output : Outport  VectorParamsAs1DForOutWhenUnconnected=off
  wires:
  Unit Delay1/1 -> Output/1
  Switch2/1 -> Unit Delay2/1
  Unit Delay2/1 -> Switch3/1
  Constant11/1 -> Switch3/3
  Switch3/1 -> CycleTrigger/1(In1)
  Constant10/1 -> Switch2/3
  Constant8/1 -> Switch2/1
  CycleTrigger/1(Trigger) -> Unit Delay1/1, Switch2/2
  Condition/1 -> Switch3/2
  TimeCount/1 -> CycleTrigger/2(In2)

== system EPT/Foreground_TimeBase_5ms/E//W /BP-OBU_E//W/BP-OBU_E//W/BP-OBU_Warning//Fault_G1/Tbp E//W/Delay12 ==
  Condition : Inport
  TimeCount : Inport  Port=2
  Constant10 : Constant
  Constant11 : Constant  Value=0
  Constant8 : Constant  Value=0
  CycleTrigger : Subsystem
  Switch2 : Switch  Threshold=1
  Switch3 : Switch  Threshold=1
  Unit Delay1 : UnitDelay  SampleTime=-1  HasFrameUpgradeWarning=on
  Unit Delay2 : UnitDelay  SampleTime=-1  HasFrameUpgradeWarning=on
  Output : Outport  VectorParamsAs1DForOutWhenUnconnected=off
  wires:
  TimeCount/1 -> CycleTrigger/2(In2)
  Condition/1 -> Switch3/2
  CycleTrigger/1(Trigger) -> Switch2/2, Unit Delay1/1
  Constant8/1 -> Switch2/1
  Constant10/1 -> Switch2/3
  Switch3/1 -> CycleTrigger/1(In1)
  Constant11/1 -> Switch3/3
  Unit Delay2/1 -> Switch3/1
  Switch2/1 -> Unit Delay2/1
  Unit Delay1/1 -> Output/1

== system EPT/Foreground_TimeBase_5ms/E//W /BP-OBU_E//W/BP-OBU_E//W/BP-OBU_Warning//Fault_G1/Tbp E//W/Delay13 ==
  Condition : Inport
  TimeCount : Inport  Port=2
  Constant10 : Constant
  Constant11 : Constant  Value=0
  Constant8 : Constant  Value=0
  CycleTrigger : Subsystem
  Switch2 : Switch  Threshold=1
  Switch3 : Switch  Threshold=1
  Unit Delay1 : UnitDelay  SampleTime=-1  HasFrameUpgradeWarning=on
  Unit Delay2 : UnitDelay  SampleTime=-1  HasFrameUpgradeWarning=on
  Output : Outport  VectorParamsAs1DForOutWhenUnconnected=off
  wires:
  Unit Delay1/1 -> Output/1
  Switch2/1 -> Unit Delay2/1
  Unit Delay2/1 -> Switch3/1
  Constant11/1 -> Switch3/3
  Switch3/1 -> CycleTrigger/1(In1)
  Constant10/1 -> Switch2/3
  Constant8/1 -> Switch2/1
  CycleTrigger/1(Trigger) -> Unit Delay1/1, Switch2/2
  Condition/1 -> Switch3/2
  TimeCount/1 -> CycleTrigger/2(In2)

== system EPT/Foreground_TimeBase_5ms/E//W /BP-OBU_E//W/BP-OBU_E//W/BP-OBU_Warning//Fault_G1/Tbp E//W/Delay14 ==
  Condition : Inport
  TimeCount : Inport  Port=2
  Constant10 : Constant
  Constant11 : Constant  Value=0
  Constant8 : Constant  Value=0
  CycleTrigger : Subsystem
  Switch2 : Switch  Threshold=1
  Switch3 : Switch  Threshold=1
  Unit Delay1 : UnitDelay  SampleTime=-1  HasFrameUpgradeWarning=on
  Unit Delay2 : UnitDelay  SampleTime=-1  HasFrameUpgradeWarning=on
  Output : Outport  VectorParamsAs1DForOutWhenUnconnected=off
  wires:
  TimeCount/1 -> CycleTrigger/2(In2)
  Condition/1 -> Switch3/2
  CycleTrigger/1(Trigger) -> Switch2/2, Unit Delay1/1
  Constant8/1 -> Switch2/1
  Constant10/1 -> Switch2/3
  Switch3/1 -> CycleTrigger/1(In1)
  Constant11/1 -> Switch3/3
  Unit Delay2/1 -> Switch3/1
  Switch2/1 -> Unit Delay2/1
  Unit Delay1/1 -> Output/1

== system EPT/Foreground_TimeBase_5ms/E//W /BP-OBU_E//W/BP-OBU_E//W/BP-OBU_Warning//Fault_G1/Tbp E//W/Delay15 ==
  Condition : Inport
  TimeCount : Inport  Port=2
  Constant10 : Constant
  Constant11 : Constant  Value=0
  Constant8 : Constant  Value=0
  CycleTrigger : Subsystem
  Switch2 : Switch  Threshold=1
  Switch3 : Switch  Threshold=1
  Unit Delay1 : UnitDelay  SampleTime=-1  HasFrameUpgradeWarning=on
  Unit Delay2 : UnitDelay  SampleTime=-1  HasFrameUpgradeWarning=on
  Output : Outport  VectorParamsAs1DForOutWhenUnconnected=off
  wires:
  Unit Delay1/1 -> Output/1
  Switch2/1 -> Unit Delay2/1
  Unit Delay2/1 -> Switch3/1
  Constant11/1 -> Switch3/3
  Switch3/1 -> CycleTrigger/1(In1)
  Constant10/1 -> Switch2/3
  Constant8/1 -> Switch2/1
  CycleTrigger/1(Trigger) -> Unit Delay1/1, Switch2/2
  Condition/1 -> Switch3/2
  TimeCount/1 -> CycleTrigger/2(In2)

== system EPT/Foreground_TimeBase_5ms/E//W /BP-OBU_E//W/BP-OBU_E//W/BP-OBU_Warning//Fault_G1/Tbp E//W/Latch10 ==
  Latch : Inport
  Reset : Inport  Port=2
  Switch1 : Switch  Criteria=u2 > Threshold
  Switch3 : Switch  Criteria=u2 > Threshold
  Unit Delay1 : UnitDelay  SampleTime=-1  HasFrameUpgradeWarning=on
  Output : Outport  VectorParamsAs1DForOutWhenUnconnected=off
  wires:
  Unit Delay1/1 -> Switch1/3
  Switch3/1 -> Output/1, Unit Delay1/1
  Reset/1 -> Switch3/2
  Latch/1 -> Switch1/1, Switch1/2
  Switch1/1 -> Switch3/3

== system EPT/Foreground_TimeBase_5ms/E//W /BP-OBU_E//W/BP-OBU_E//W/BP-OBU_Warning//Fault_G1/Tbp E//W/Latch11 ==
  Latch : Inport
  Reset : Inport  Port=2
  Switch1 : Switch  Criteria=u2 > Threshold
  Switch3 : Switch  Criteria=u2 > Threshold
  Unit Delay1 : UnitDelay  SampleTime=-1  HasFrameUpgradeWarning=on
  Output : Outport  VectorParamsAs1DForOutWhenUnconnected=off
  wires:
  Switch1/1 -> Switch3/3
  Latch/1 -> Switch1/2, Switch1/1
  Reset/1 -> Switch3/2
  Switch3/1 -> Unit Delay1/1, Output/1
  Unit Delay1/1 -> Switch1/3

== system EPT/Foreground_TimeBase_5ms/E//W /BP-OBU_E//W/BP-OBU_E//W/BP-OBU_Warning//Fault_G1/Tbp E//W/Latch12 ==
  Latch : Inport
  Reset : Inport  Port=2
  Switch1 : Switch  Criteria=u2 > Threshold
  Switch3 : Switch  Criteria=u2 > Threshold
  Unit Delay1 : UnitDelay  SampleTime=-1  HasFrameUpgradeWarning=on
  Output : Outport  VectorParamsAs1DForOutWhenUnconnected=off
  wires:
  Unit Delay1/1 -> Switch1/3
  Switch3/1 -> Output/1, Unit Delay1/1
  Reset/1 -> Switch3/2
  Latch/1 -> Switch1/1, Switch1/2
  Switch1/1 -> Switch3/3

== system EPT/Foreground_TimeBase_5ms/E//W /BP-OBU_E//W/BP-OBU_E//W/BP-OBU_Warning//Fault_G1/Tbp E//W/Latch13 ==
  Latch : Inport
  Reset : Inport  Port=2
  Switch1 : Switch  Criteria=u2 > Threshold
  Switch3 : Switch  Criteria=u2 > Threshold
  Unit Delay1 : UnitDelay  SampleTime=-1  HasFrameUpgradeWarning=on
  Output : Outport  VectorParamsAs1DForOutWhenUnconnected=off
  wires:
  Switch1/1 -> Switch3/3
  Latch/1 -> Switch1/2, Switch1/1
  Reset/1 -> Switch3/2
  Switch3/1 -> Unit Delay1/1, Output/1
  Unit Delay1/1 -> Switch1/3

== system EPT/Foreground_TimeBase_5ms/E//W /BP-OBU_E//W/BP-OBU_E//W/BP-OBU_Warning//Fault_G1/Tbp E//W/Latch14 ==
  Latch : Inport
  Reset : Inport  Port=2
  Switch1 : Switch  Criteria=u2 > Threshold
  Switch3 : Switch  Criteria=u2 > Threshold
  Unit Delay1 : UnitDelay  SampleTime=-1  HasFrameUpgradeWarning=on
  Output : Outport  VectorParamsAs1DForOutWhenUnconnected=off
  wires:
  Unit Delay1/1 -> Switch1/3
  Switch3/1 -> Output/1, Unit Delay1/1
  Reset/1 -> Switch3/2
  Latch/1 -> Switch1/1, Switch1/2
  Switch1/1 -> Switch3/3

== system EPT/Foreground_TimeBase_5ms/E//W /BP-OBU_E//W/BP-OBU_E//W/BP-OBU_Warning//Fault_G1/Tbp E//W/Latch15 ==
  Latch : Inport
  Reset : Inport  Port=2
  Switch1 : Switch  Criteria=u2 > Threshold
  Switch3 : Switch  Criteria=u2 > Threshold
  Unit Delay1 : UnitDelay  SampleTime=-1  HasFrameUpgradeWarning=on
  Output : Outport  VectorParamsAs1DForOutWhenUnconnected=off
  wires:
  Switch1/1 -> Switch3/3
  Latch/1 -> Switch1/2, Switch1/1
  Reset/1 -> Switch3/2
  Switch3/1 -> Unit Delay1/1, Output/1
  Unit Delay1/1 -> Switch1/3

== system EPT/Foreground_TimeBase_5ms/E//W /BP-OBU_E//W/BP-OBU_E//W/BP-OBU_Warning//Fault_G1/Vbp E//W/Delay ==
  Condition : Inport
  TimeCount : Inport  Port=2
  Constant10 : Constant
  Constant11 : Constant  Value=0
  Constant8 : Constant  Value=0
  CycleTrigger : Subsystem
  Switch2 : Switch  Threshold=1
  Switch3 : Switch  Threshold=1
  Unit Delay1 : UnitDelay  SampleTime=-1  HasFrameUpgradeWarning=on
  Unit Delay2 : UnitDelay  SampleTime=-1  HasFrameUpgradeWarning=on
  Output : Outport  VectorParamsAs1DForOutWhenUnconnected=off
  wires:
  TimeCount/1 -> CycleTrigger/2(In2)
  Condition/1 -> Switch3/2
  CycleTrigger/1(Trigger) -> Switch2/2, Unit Delay1/1
  Constant8/1 -> Switch2/1
  Constant10/1 -> Switch2/3
  Switch3/1 -> CycleTrigger/1(In1)
  Constant11/1 -> Switch3/3
  Unit Delay2/1 -> Switch3/1
  Switch2/1 -> Unit Delay2/1
  Unit Delay1/1 -> Output/1

== system EPT/Foreground_TimeBase_5ms/E//W /BP-OBU_E//W/BP-OBU_E//W/BP-OBU_Warning//Fault_G1/Vbp E//W/Delay1 ==
  Condition : Inport
  TimeCount : Inport  Port=2
  Constant10 : Constant
  Constant11 : Constant  Value=0
  Constant8 : Constant  Value=0
  CycleTrigger : Subsystem
  Switch2 : Switch  Threshold=1
  Switch3 : Switch  Threshold=1
  Unit Delay1 : UnitDelay  SampleTime=-1  HasFrameUpgradeWarning=on
  Unit Delay2 : UnitDelay  SampleTime=-1  HasFrameUpgradeWarning=on
  Output : Outport  VectorParamsAs1DForOutWhenUnconnected=off
  wires:
  Unit Delay1/1 -> Output/1
  Switch2/1 -> Unit Delay2/1
  Unit Delay2/1 -> Switch3/1
  Constant11/1 -> Switch3/3
  Switch3/1 -> CycleTrigger/1(In1)
  Constant10/1 -> Switch2/3
  Constant8/1 -> Switch2/1
  CycleTrigger/1(Trigger) -> Unit Delay1/1, Switch2/2
  Condition/1 -> Switch3/2
  TimeCount/1 -> CycleTrigger/2(In2)

== system EPT/Foreground_TimeBase_5ms/E//W /BP-OBU_E//W/BP-OBU_E//W/BP-OBU_Warning//Fault_G1/Vbp E//W/Delay2 ==
  Condition : Inport
  TimeCount : Inport  Port=2
  Constant10 : Constant
  Constant11 : Constant  Value=0
  Constant8 : Constant  Value=0
  CycleTrigger : Subsystem
  Switch2 : Switch  Threshold=1
  Switch3 : Switch  Threshold=1
  Unit Delay1 : UnitDelay  SampleTime=-1  HasFrameUpgradeWarning=on
  Unit Delay2 : UnitDelay  SampleTime=-1  HasFrameUpgradeWarning=on
  Output : Outport  VectorParamsAs1DForOutWhenUnconnected=off
  wires:
  TimeCount/1 -> CycleTrigger/2(In2)
  Condition/1 -> Switch3/2
  CycleTrigger/1(Trigger) -> Switch2/2, Unit Delay1/1
  Constant8/1 -> Switch2/1
  Constant10/1 -> Switch2/3
  Switch3/1 -> CycleTrigger/1(In1)
  Constant11/1 -> Switch3/3
  Unit Delay2/1 -> Switch3/1
  Switch2/1 -> Unit Delay2/1
  Unit Delay1/1 -> Output/1

== system EPT/Foreground_TimeBase_5ms/E//W /BP-OBU_E//W/BP-OBU_E//W/BP-OBU_Warning//Fault_G1/Vbp E//W/Delay3 ==
  Condition : Inport
  TimeCount : Inport  Port=2
  Constant10 : Constant
  Constant11 : Constant  Value=0
  Constant8 : Constant  Value=0
  CycleTrigger : Subsystem
  Switch2 : Switch  Threshold=1
  Switch3 : Switch  Threshold=1
  Unit Delay1 : UnitDelay  SampleTime=-1  HasFrameUpgradeWarning=on
  Unit Delay2 : UnitDelay  SampleTime=-1  HasFrameUpgradeWarning=on
  Output : Outport  VectorParamsAs1DForOutWhenUnconnected=off
  wires:
  Unit Delay1/1 -> Output/1
  Switch2/1 -> Unit Delay2/1
  Unit Delay2/1 -> Switch3/1
  Constant11/1 -> Switch3/3
  Switch3/1 -> CycleTrigger/1(In1)
  Constant10/1 -> Switch2/3
  Constant8/1 -> Switch2/1
  CycleTrigger/1(Trigger) -> Unit Delay1/1, Switch2/2
  Condition/1 -> Switch3/2
  TimeCount/1 -> CycleTrigger/2(In2)

== system EPT/Foreground_TimeBase_5ms/E//W /BP-OBU_E//W/BP-OBU_E//W/BP-OBU_Warning//Fault_G1/Vbp E//W/Latch ==
  Latch : Inport
  Reset : Inport  Port=2
  Switch1 : Switch  Criteria=u2 > Threshold
  Switch3 : Switch  Criteria=u2 > Threshold
  Unit Delay1 : UnitDelay  SampleTime=-1  HasFrameUpgradeWarning=on
  Output : Outport  VectorParamsAs1DForOutWhenUnconnected=off
  wires:
  Unit Delay1/1 -> Switch1/3
  Switch3/1 -> Output/1, Unit Delay1/1
  Reset/1 -> Switch3/2
  Latch/1 -> Switch1/1, Switch1/2
  Switch1/1 -> Switch3/3

== system EPT/Foreground_TimeBase_5ms/E//W /BP-OBU_E//W/BP-OBU_E//W/BP-OBU_Warning//Fault_G1/Vbp E//W/Latch1 ==
  Latch : Inport
  Reset : Inport  Port=2
  Switch1 : Switch  Criteria=u2 > Threshold
  Switch3 : Switch  Criteria=u2 > Threshold
  Unit Delay1 : UnitDelay  SampleTime=-1  HasFrameUpgradeWarning=on
  Output : Outport  VectorParamsAs1DForOutWhenUnconnected=off
  wires:
  Switch1/1 -> Switch3/3
  Latch/1 -> Switch1/2, Switch1/1
  Reset/1 -> Switch3/2
  Switch3/1 -> Unit Delay1/1, Output/1
  Unit Delay1/1 -> Switch1/3

== system EPT/Foreground_TimeBase_5ms/E//W /BP-OBU_E//W/BP-OBU_E//W/BP-OBU_Warning//Fault_G1/Vbp E//W/Latch2 ==
  Latch : Inport
  Reset : Inport  Port=2
  Switch1 : Switch  Criteria=u2 > Threshold
  Switch3 : Switch  Criteria=u2 > Threshold
  Unit Delay1 : UnitDelay  SampleTime=-1  HasFrameUpgradeWarning=on
  Output : Outport  VectorParamsAs1DForOutWhenUnconnected=off
  wires:
  Unit Delay1/1 -> Switch1/3
  Switch3/1 -> Output/1, Unit Delay1/1
  Reset/1 -> Switch3/2
  Latch/1 -> Switch1/1, Switch1/2
  Switch1/1 -> Switch3/3

== system EPT/Foreground_TimeBase_5ms/E//W /BP-OBU_E//W/BP-OBU_E//W/BP-OBU_Warning//Fault_G1/Vbp E//W/Latch3 ==
  Latch : Inport
  Reset : Inport  Port=2
  Switch1 : Switch  Criteria=u2 > Threshold
  Switch3 : Switch  Criteria=u2 > Threshold
  Unit Delay1 : UnitDelay  SampleTime=-1  HasFrameUpgradeWarning=on
  Output : Outport  VectorParamsAs1DForOutWhenUnconnected=off
  wires:
  Switch1/1 -> Switch3/3
  Latch/1 -> Switch1/2, Switch1/1
  Reset/1 -> Switch3/2
  Switch3/1 -> Unit Delay1/1, Output/1
  Unit Delay1/1 -> Switch1/3

== system EPT/Foreground_TimeBase_5ms/E//W /BP-OBU_E//W/BP-OBU_E//W/BP-OBU_Warning//Fault_G2/Tcell E//W/Delay1 ==
  Condition : Inport
  TimeCount : Inport  Port=2
  Constant10 : Constant
  Constant11 : Constant  Value=0
  Constant8 : Constant  Value=0
  CycleTrigger : Subsystem
  Switch2 : Switch  Threshold=1
  Switch3 : Switch  Threshold=1
  Unit Delay1 : UnitDelay  SampleTime=-1  HasFrameUpgradeWarning=on
  Unit Delay2 : UnitDelay  SampleTime=-1  HasFrameUpgradeWarning=on
  Output : Outport  VectorParamsAs1DForOutWhenUnconnected=off
  wires:
  Unit Delay1/1 -> Output/1
  Switch2/1 -> Unit Delay2/1
  Unit Delay2/1 -> Switch3/1
  Constant11/1 -> Switch3/3
  Switch3/1 -> CycleTrigger/1(In1)
  Constant10/1 -> Switch2/3
  Constant8/1 -> Switch2/1
  CycleTrigger/1(Trigger) -> Unit Delay1/1, Switch2/2
  Condition/1 -> Switch3/2
  TimeCount/1 -> CycleTrigger/2(In2)

== system EPT/Foreground_TimeBase_5ms/E//W /BP-OBU_E//W/BP-OBU_E//W/BP-OBU_Warning//Fault_G2/Tcell E//W/Delay2 ==
  Condition : Inport
  TimeCount : Inport  Port=2
  Constant10 : Constant
  Constant11 : Constant  Value=0
  Constant8 : Constant  Value=0
  CycleTrigger : Subsystem
  Switch2 : Switch  Threshold=1
  Switch3 : Switch  Threshold=1
  Unit Delay1 : UnitDelay  SampleTime=-1  HasFrameUpgradeWarning=on
  Unit Delay2 : UnitDelay  SampleTime=-1  HasFrameUpgradeWarning=on
  Output : Outport  VectorParamsAs1DForOutWhenUnconnected=off
  wires:
  TimeCount/1 -> CycleTrigger/2(In2)
  Condition/1 -> Switch3/2
  CycleTrigger/1(Trigger) -> Switch2/2, Unit Delay1/1
  Constant8/1 -> Switch2/1
  Constant10/1 -> Switch2/3
  Switch3/1 -> CycleTrigger/1(In1)
  Constant11/1 -> Switch3/3
  Unit Delay2/1 -> Switch3/1
  Switch2/1 -> Unit Delay2/1
  Unit Delay1/1 -> Output/1

== system EPT/Foreground_TimeBase_5ms/E//W /BP-OBU_E//W/BP-OBU_E//W/BP-OBU_Warning//Fault_G2/Tcell E//W/Delay22 ==
  Condition : Inport
  TimeCount : Inport  Port=2
  Constant10 : Constant
  Constant11 : Constant  Value=0
  Constant8 : Constant  Value=0
  CycleTrigger : Subsystem
  Switch2 : Switch  Threshold=1
  Switch3 : Switch  Threshold=1
  Unit Delay1 : UnitDelay  SampleTime=-1  HasFrameUpgradeWarning=on
  Unit Delay2 : UnitDelay  SampleTime=-1  HasFrameUpgradeWarning=on
  Output : Outport  VectorParamsAs1DForOutWhenUnconnected=off
  wires:
  TimeCount/1 -> CycleTrigger/2(In2)
  Condition/1 -> Switch3/2
  CycleTrigger/1(Trigger) -> Switch2/2, Unit Delay1/1
  Constant8/1 -> Switch2/1
  Constant10/1 -> Switch2/3
  Switch3/1 -> CycleTrigger/1(In1)
  Constant11/1 -> Switch3/3
  Unit Delay2/1 -> Switch3/1
  Switch2/1 -> Unit Delay2/1
  Unit Delay1/1 -> Output/1

== system EPT/Foreground_TimeBase_5ms/E//W /BP-OBU_E//W/BP-OBU_E//W/BP-OBU_Warning//Fault_G2/Tcell E//W/Delay3 ==
  Condition : Inport
  TimeCount : Inport  Port=2
  Constant10 : Constant
  Constant11 : Constant  Value=0
  Constant8 : Constant  Value=0
  CycleTrigger : Subsystem
  Switch2 : Switch  Threshold=1
  Switch3 : Switch  Threshold=1
  Unit Delay1 : UnitDelay  SampleTime=-1  HasFrameUpgradeWarning=on
  Unit Delay2 : UnitDelay  SampleTime=-1  HasFrameUpgradeWarning=on
  Output : Outport  VectorParamsAs1DForOutWhenUnconnected=off
  wires:
  Unit Delay1/1 -> Output/1
  Switch2/1 -> Unit Delay2/1
  Unit Delay2/1 -> Switch3/1
  Constant11/1 -> Switch3/3
  Switch3/1 -> CycleTrigger/1(In1)
  Constant10/1 -> Switch2/3
  Constant8/1 -> Switch2/1
  CycleTrigger/1(Trigger) -> Unit Delay1/1, Switch2/2
  Condition/1 -> Switch3/2
  TimeCount/1 -> CycleTrigger/2(In2)
